simulink model "usart1TestRcvChar"  (R2015b)
settings: Solver=FixedStepDiscrete  StartTime=0.0  StopTime=10.0  RelTol=1e-3
libraries: USART_Lib x2, GPIO_Lib x1, STM32_Config_Lib x1
settings Model: Creator=reynaudp  LastModifiedBy=reynaudp
settings DataIOCC: SaveFormat=Array  SignalLoggingSaveFormat=ModelDataLogs
settings OptimizationCC: OptimizeModelRefInitCode=on  LifeSpan=1
settings DebuggingCC: UnderspecifiedInitializationDetection=Classic  MergeDetectMultiDrivingBlocksExec=none  SolverPrmCheckMsg=warning  MultiTaskDSMMsg=warning  MultiTaskCondExecSysMsg=none
settings HardwareCC: ProdBitPerPointer=32  ProdLargestAtomicInteger=Integer  ProdWordSize=32  ProdHWDeviceType=STMicroelectronics->STM32 32-bit Cortex-M
settings RTWCC: SystemTargetFile=stm32.tlc  TemplateMakefile=stm32.tmf  Description=stm32 (Embedded Target)  GenerateReport=on  LaunchReport=on
settings CodeAppCC: IgnoreCustomStorageClasses=off  MaxIdLength=64  CustomSymbolStrType=$N$R$M  SimulinkBlockComments=off
settings STFCustomTargetCC: CodeReplacementLibrary=ARM CMSIS SIN COS  ParMdlRefBuildCompliant=on  ConcurrentExecutionCompliant=off  IncludeMdlTerminateFcn=off  GeneratePreprocessorConditionals=Use local settings  CombineOutputUpdateFcns=on  ERTCustomFileBanners=on  SupportContinuousTime=off  SupportNonInlinedSFcns=off  MATLABClassNameForMDSCustomization=Simulink.SoftwareTarget.ERTCustomization  CPPClassGenCompliant=off  GRTInterface=off  SystemTargetFile=stm32.tlc
settings ERTTargetCC: CodeReplacementLibrary=ARM CMSIS SIN COS  CompOptLevelCompliant=off  ConcurrentExecutionCompliant=off  IncludeMdlTerminateFcn=off  ERTFirstTimeCompliant=off  ModelStepFunctionPrototypeControlCompliant=off  CPPClassGenCompliant=off  UseToolchainInfoCompliant=off  ERTSrcFileBannerTemplate=sourceFileTemplate.cgt  ERTHdrFileBannerTemplate=sourceFileTemplate.cgt  ERTDataSrcFileTemplate=sourceFileTemplate.cgt  ERTDataHdrFileTemplate=sourceFileTemplate.cgt  ERTCustomFileTemplate=customRoutineProcess.tlc
settings ConfigComp: CovModelRefEnable=Off  CovSFcnEnable=off

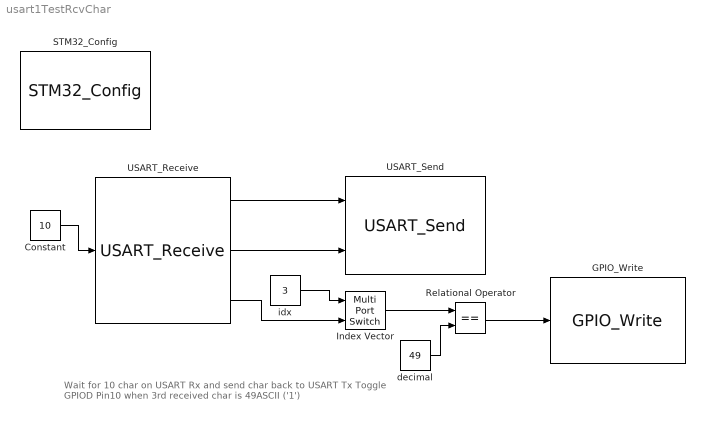
== system usart1TestRcvChar ==
  note: Wait for 10 char on USART Rx and send char back to USART Tx
      | Toggle GPIOD Pin10 when 3rd received char is 49ASCII ('1')
  Constant : Constant  Value=10  OutDataTypeStr=uint16
  GPIO_Write : GPIO_Lib/GPIO_Write  Port_name=GPIOD  Pin0=off  Toggle_Pin0=off  Pin1=off  Toggle_Pin1=off  Pin2=off  Toggle_Pin2=off  Pin3=off  Toggle_Pin3=off  Pin4=off  Toggle_Pin4=off  Pin5=off  Toggle_Pin5=off  Pin6=off  Toggle_Pin6=off  Pin7=off  Toggle_Pin7=off  Pin8=off  Toggle_Pin8=off  Pin9=off  Toggle_Pin9=off  Pin10=on  Toggle_Pin10=off  Pin11=off  Toggle_Pin11=off  Pin12=off  Toggle_Pin12=off  Pin13=off  Toggle_Pin13=off  Pin14=off  Toggle_Pin14=off  Pin15=off  Toggle_Pin15=off  PinList=GPIOD10
  Index Vector : MultiPortSwitch  DataPortOrder=Zero-based contiguous  Inputs=1  zeroidx=on  OutDataTypeStr=uint8
  Relational Operator : RelationalOperator  Operator===  OutDataTypeStr=boolean
  STM32_Config : STM32_Config_Lib/STM32_Config  Priority=0  Project_Path=.\  Config_File=usart1TestRcvChar.ioc  MCU_Name=STM32F407VGTx
  USART_Receive : USART_Lib/USART_Receive  USART_name=USART1  Buff_size=32  nbUsart=1  Soft_it=off  Soft_num=0  usartMode=Asynchronous  usartDma_Rx=off  usartDma_Tx=off  usartIt=on
  USART_Send : USART_Lib/USART_Send  USART_name=USART1  Buff_size=128  nbUsart=1  usartMode=Asynchronous  usartDma_Rx=off  usartDma_Tx=off  usartIt=on
  decimal : Constant  Value=49  OutDataTypeStr=uint8
  idx : Constant  Value=3  OutDataTypeStr=uint8
  wires:
  Constant/1 -> USART_Receive/1
  USART_Receive/1 -> USART_Send/1
  USART_Receive/2 -> USART_Send/2
  USART_Receive/3 -> Index Vector/2
  idx/1 -> Index Vector/1
  Index Vector/1 -> Relational Operator/1
  decimal/1 -> Relational Operator/2
  Relational Operator/1 -> GPIO_Write/1
